simulink model "LR_2_var15 (1)"  (R2020b)
settings: Solver=VariableStepAuto  StartTime=0.0  StopTime=160  RelTol=1e-3
libraries: simulink x2
settings Model: Creator=SIA  LastModifiedBy=SIA

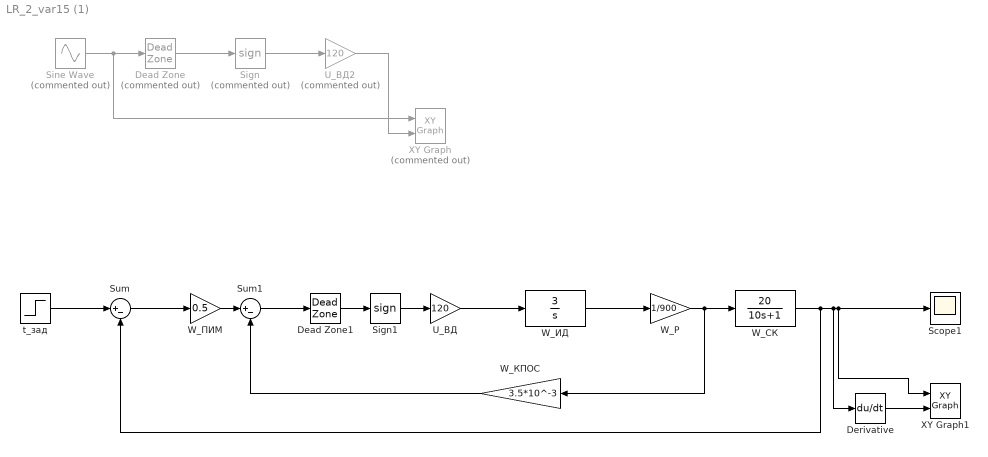
== system LR_2_var15 (1) ==
  Dead Zone : DeadZone  Commented=on  LowerValue=-0.3  UpperValue=0.3  SaturateOnIntegerOverflow=on
  Dead Zone1 : DeadZone  LowerValue=-0.3  UpperValue=0.3  SaturateOnIntegerOverflow=on
  Derivative : Derivative
  Scope1 : Scope
  Sign : Signum  Commented=on
  Sign1 : Signum
  Sine Wave : Sin  Commented=on  SampleTime=0
  Sum : Sum  Inputs=|+-
  Sum1 : Sum  Inputs=|+-
  U_ВД : Gain  Gain=120
  U_ВД2 : Gain  Commented=on  Gain=120
  W_ИД : TransferFcn  Numerator=[3]  Denominator=[1 0]
  W_КПОС : Gain  Gain=3.5*10^-3
  W_ПИМ : Gain  Gain=0.5
  W_Р : Gain  Gain=1/900
  W_СК : TransferFcn  Numerator=[20]  Denominator=[10 1]
  XY Graph : simulink/Sinks/XY Graph  Commented=on  xmin=-1  xmax=1  ymin=-125  ymax=125  st=-1
  XY Graph1 : simulink/Sinks/XY Graph  xmin=-10  xmax=130  ymin=-6  ymax=7.2  st=0.1
  t_зад : Step  Time=0  After=100  SampleTime=0
  wires:
  Sign/1 -> U_ВД2/1
  Dead Zone/1 -> Sign/1
  Sine Wave/1 -> XY Graph/1, Dead Zone/1
  U_ВД2/1 -> XY Graph/2
  Sum/1 -> W_ПИМ/1
  Dead Zone1/1 -> Sign1/1
  Sign1/1 -> U_ВД/1
  W_ПИМ/1 -> Sum1/1
  Sum1/1 -> Dead Zone1/1
  U_ВД/1 -> W_ИД/1
  W_ИД/1 -> W_Р/1
  W_Р/1 -> W_КПОС/1, W_СК/1
  W_КПОС/1 -> Sum1/2
  t_зад/1 -> Sum/1
  Derivative/1 -> XY Graph1/2
  W_СК/1 -> Sum/2, Derivative/1, XY Graph1/1, Scope1/1
